simulink library "DevLib"  (R2013b)
settings: Solver=ode45  StartTime=0.0  StopTime=10.0  RelTol=1e-3
undefined symbols (not defined in the file): magnitude, X1, X2, Y1
libraries: simulink x12
settings Model: Creator=HZ69BY  LastModifiedBy=DZ1YRM

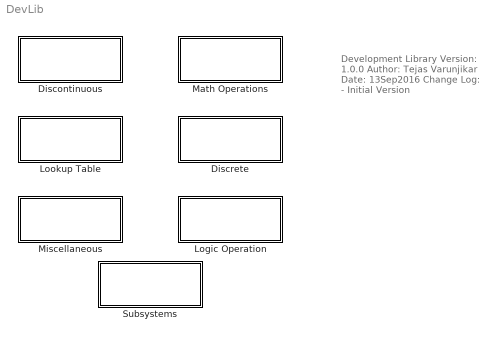
== system DevLib ==
  note: Development Library
      |
      | Version: 1.0.0
      | Author: Tejas Varunjikar
      | Date: 13Sep2016
      | Change Log:
      | - Initial Version
  Discontinuous : Subsystem  mask(Discontinuous){}
      mask Display: fprintf('Discontinuous')
  Discrete : Subsystem
      mask Display: fprintf('Discrete');
  Logic Operation : Subsystem  mask(Logic Operations){}
      mask Display: fprintf('Logic Operation')
  Lookup Table : Subsystem  mask(Lookup Tables){}
      mask Display: fprintf('LookupTable');
  Math Operations : Subsystem  mask(Math Operations){}
      mask Display: fprintf('MathOperations')
  Miscellaneous : Subsystem  mask(Miscellaneous){}
      mask Display: fprintf('Miscellaneous')
  "Subsystems " : Subsystem  mask(Subsystems){}
      mask Display: fprintf('Subsystems')

== system DevLib/Discontinuous ==
  Dead Zone : DeadZone  SaturateOnIntegerOverflow=on
  Dead Zone Dynamic : simulink/Discontinuities/Dead Zone Dynamic
  Rate Limiter : RateLimiter  SampleTimeMode=inherited
  Rate Limiter Dynamic : simulink/Discontinuities/Rate Limiter Dynamic
  Saturation : Saturate
  Saturation Dynamic : simulink/Discontinuities/Saturation Dynamic  OutMin=[]  OutMax=[]  OutDataTypeStr=Inherit: Same as second input  OutDataType=fixdt(1, 16)  OutScaling=2^-10  DoSatur=off

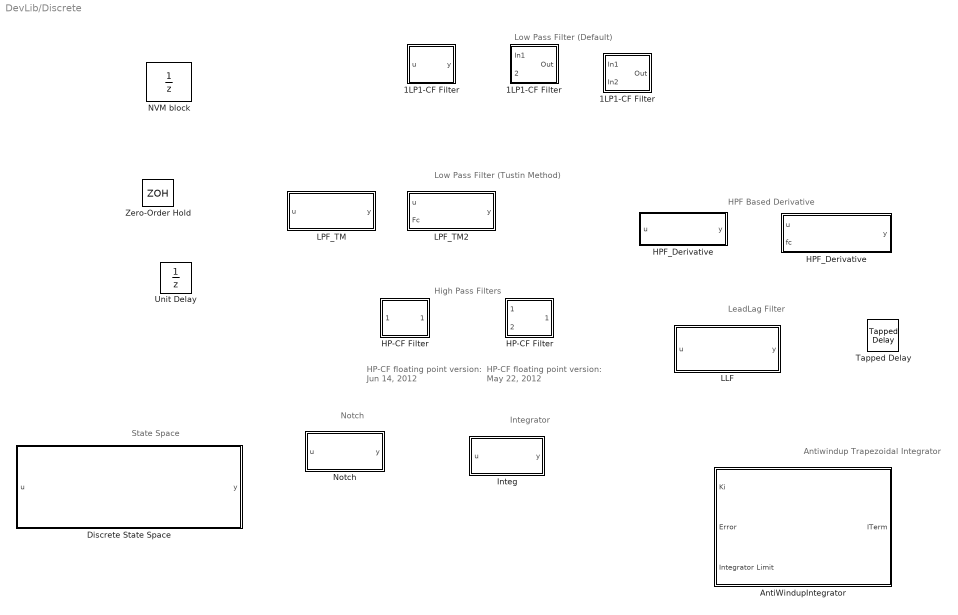
== system DevLib/Discrete ==
  note: HP-CF floating point
      | version:  Jun 14, 2012
  note: HP-CF floating point
      | version:  May 22, 2012
  note: Low Pass Filter (Default)
  note: High Pass Filters
  note: Low Pass Filter (Tustin Method)
  note: Notch
  note: HPF Based Derivative
  note: LeadLag Filter
  note: Integrator
  note: Antiwindup Trapezoidal Integrator
  note: State Space
  " 1LP1-CF Filter " : Subsystem  mask(1LP1-CF Filter){Ts=.002, IC=0}
      mask prompts: Ts "Function Time Step (seconds)"; IC "Initial Condition (Enineering Units)"
      mask help: version: May 22, 2012
      mask Display:
      | port_label('input',1,'u')
      | port_label('input',2,'Hz')
      | port_label('output',1,'y')
      | 
      | %a = [2:0.1:5.2]';
      | %b = sin(2*a);
      | %c = 0.7*sin(25*a);
      | %d = b+c;
      | %e = vertcat(d, b);
      | %plot(e);
      | 
      | disp 'LPF'
  1LP1-CF Filter : Subsystem  mask(1LP1-CF Filter){Ts=.002, Kn_Hz=30, IC=0}
      mask prompts: Ts "Function Time Step (seconds)"; Kn_Hz "Cutoff Frequency in Hz"; IC "Initial Condition (Enineering Units)"
      mask help: version: Jun 14, 2012
      mask init:
      | %Convert cutoff frequency from Hz into floating point "counts"
      | Kn_Cnt = 1-exp(-2*pi*Kn_Hz*Ts);
      | 
      | %Filter design document originally called this value Knum
      | Knum = Kn_Cnt;
      mask Display:
      | port_label('input',1,'u')
      | port_label('output',1,'y')
      | disp 'LPF'
      | 
      | %a = [2:0.1:5.2]';
      | %b = sin(2*a);
      | %c = 0.7*sin(25*a);
      | %d = b+c;
      | %e = vertcat(d, b);
      | %plot(e);
  "1LP1-CF Filter " : Subsystem  mask(1LP1-CF Filter){Ts=.002, Kn_Hz=30}
      mask prompts: Ts "Function Time Step (seconds)"; Kn_Hz "Cutoff Frequency in Hz"
      mask help: version: Aug 31, 2012
      mask init:
      | %Convert cutoff frequency from Hz into floating point "counts"
      | Kn_Cnt = 1-exp(-2*pi*Kn_Hz*Ts);
      | 
      | %Filter design document originally called this value Knum
      | Knum = Kn_Cnt;
      mask Help:
      | 1st order floating point low-pass filter, designated within Nexteer as 1LP1-CF.
      | 
      | This block is arranged to use an externally supplied state variable.  The filter
      | is initialized to the state variable's I.C.
      mask Display:
      | port_label('input',1,'u')
      | port_label('input',2,'sv')
      | port_label('output',1,'y')
      | 
      | disp 'LPF'
  AntiWindupIntegrator : Subsystem  mask(Antiwindup Integrator){Ts=0.002, AntiWdupGain=0}
      mask prompts: Ts "Sample Time"; AntiWdupGain "Anti windup Gain"
      mask help: This is a standard antiwindup integrator design typically used.
      mask Display:
      | fprintf('Antiwindup Integrator');
      | port_label('input',1,'Ki')
      | port_label('input',2,'Error')
      | port_label('input',3,'Integrator Limit')
      | port_label('output',1,'I_term')
  Discrete State Space : Subsystem  mask(Discrete State Space){MtrxA=1, MtrxB=1, MtrxC=1, MtrxD=0, Ts=0.002}
      mask prompts: MtrxA "A"; MtrxB "B"; MtrxC "C"; MtrxD "D"
      mask help:
      | Discrete State Space block representation. Please enter value of state-space matrices. Input, u, is the actuation input to the plant and output, y, is measured state (plant) or estimated state (observer).
      | Input (u) and output (y) could be vectors or single numbers.
      mask Display:
      | fprintf('Discrete State Space');
      | port_label('input',1,'Input')
      | port_label('output',1,'Output')
  HP-CF Filter : Subsystem  mask(HP-CF Filter){Ts_sec=0.002, Fc_Hz=50, LP_IC=0}
      mask prompts: Ts_sec "Function Time Step (seconds)"; Fc_Hz "Cutoff Frequency in Hz"; LP_IC "Input Signal Initial Condition (Engineering Units)"
      mask help: version: June 14, 2012
      mask init:
      | % Correction factor (to be multiplied with HP part)
      | g=2*pi*Fc_Hz*Ts_sec;
      | K=sqrt(1+(2*Fc_Hz*Ts_sec)^2);
      | 
      | corr_factor=(1+exp(g))/(2*K);
      mask Display:
      | port_label('input',1,'y')
      | disp 'HPF'
      | 
      | %a = [2:0.1:5.2]';
      | %b = sin(2*a);
      | %c = 0.5*sin(25*a);
      | %d = b+c;
      | %e = vertcat(d, c);
      | %plot(e);
  "HP-CF Filter " : Subsystem  mask(HP-CF Filter){Ts_sec=0.002, LP_IC=0}
      mask prompts: Ts_sec "Function Time Step (seconds)"; LP_IC "Input Signal Initial Condition (Engineering Units)"
      mask help: version: May 22, 2012
      mask init:
      | g = 2*pi*Ts_sec;
      mask Display:
      | port_label('input',1,'y')
      | port_label('input',2,'Hz')
      | 
      | %a = [2:0.1:5.2]';
      | %b = sin(2*a);
      | %c = 0.5*sin(25*a);
      | %d = b+c;
      | %e = vertcat(d, c);
      | %plot(e);
      | 
      | disp 'HPF'
  HPF_Derivative : Subsystem  mask(High Pass Filter Derivative){Fc=10, Ts=0.002}
      mask prompts: Fc "Cutoff Frequency (Hz)"; Ts "Sample Time"
      mask init:
      | TermN=1-Ts*pi*Fc;
      | TermD=1/(1+Ts*pi*Fc);
      | UnityTerm=2*pi*Fc;
      mask Display: fprintf('HPF Derivative')
  "HPF_Derivative " : Subsystem  mask(HPF Derivative){Ts=0.002}
      mask prompts: Ts "Sample Time"
      mask help: Version June 2, 2016
      mask Display:
      | fprintf('HPF Derivative');
      | port_label('input',1,'u')
      | port_label('input',2,'Fc')
      | port_label('output',1,'y')
  Integ : Subsystem  mask(Integrator){Ki=1, Ts=0.002}
      mask prompts: Ki "Integrator Gain"; Ts "Sample Time"
      mask help:
      | Version: June 2, 2016
      | Digital integrator block representing transfer function Ki/s.
      | Ki is integrator gain.
      mask init:
      | % Initial value of a 1/z variable
      | init1=0;
      mask Display: fprintf('Integrator');
  LLF : Subsystem  mask(Lead Lag Filter){B0=0, B1=0, A1=1, Ts=0.002, Init=0}
      mask prompts: Ts "Sample Time"; Init "State Initialization"
      mask help:
      | Version: June 2, 2016
      | Filter coefficients (B0,B1,A1) of a Lead Lag Filter.
      mask Display:
      | port_label('input',1,'u')
      | port_label('output',1,'y')
      | disp 'LLF'
  LPF_TM : Subsystem  mask{Ts=0.002, fc=1}
      mask prompts: Ts "Sample Time"; fc "Cutoff Frequency"
      mask help:
      | This is a special type of Low Pass Filter.
      | It is designed using tustin transformation method.
      mask Display:
      | fprintf('LPF #2');
      | port_label('input',1,'u')
      | port_label('output',1,'y')
  "LPF_TM2 " : Subsystem  mask{Ts=0.002}
      mask prompts: Ts "Sample Time"
      mask help:
      | This is a special type of Low Pass Filter.
      | It is designed using tustin transformation method.
      mask init:
      | init1=0;
      | init2=0;
      mask Display:
      | fprintf('LPF #2');
      | port_label('input',1,'u')
      | port_label('input',2,'Fc')
      | port_label('output',1,'y')
  NVM block : UnitDelay  SampleTime=-1
      mask help: NVM (Non-volatile memory) block stores a state through ignition cycles.
      mask Display: fprintf('NVM');
  Notch : Subsystem  mask(Notch Filter){A1=0, A2=0, B0=1, B1=0, B2=0, Ts=0.002}
      mask prompts: Ts "Sample time"
      mask help:
      | version: June 2, 2016
      | Numerator (B0,B1,B2) and denominator (1,A1,A2) coefficients of 2nd order digital filter.
      mask init:
      | %Initial values of 2 1/z variables.
      | init1=0;
      | init2=0;
      mask Display: fprintf('Notch Filter')
  Tapped Delay : simulink/Discrete/Tapped Delay  vinit=0.0  samptime=-1  NumDelays=4  DelayOrder=Oldest  includeCurrent=off
  Unit Delay : UnitDelay  SampleTime=-1
  Zero-Order Hold : ZeroOrderHold

== system DevLib/Logic Operation ==
  note: Note: Various logical operators (AND, OR,.. etc. with multiple inputs allowed).
  Action Subsystem : Subsystem  TreatAsAtomicUnit=on
  Bitwise Operator : simulink/Logic and Bit Operations/Bitwise Operator  logicop=AND  UseBitMask=on  BitMask=bin2dec('11011001')  BitMaskRealWorld=Stored Integer
  Compare To Constant : simulink/Logic and Bit Operations/Compare To Constant  relop=<=  const=3.0  OutDataTypeStr=boolean
  Compare To Zero : simulink/Logic and Bit Operations/Compare To Zero  relop=<=  OutDataTypeStr=boolean
  For Iterator Subsystem : Subsystem  TreatAsAtomicUnit=on
  If : If  NumInputs=2  IfExpression=u1  ElseIfExpressions=u2
  Logical Operator : Logic  AllPortsSameDT=off  OutDataTypeStr=boolean
  Merge : Merge  Inputs=3
  Pass through Action Subsystem : Subsystem  TreatAsAtomicUnit=on  mask(pass thru, version Nov 30, 2012){nIn=1}
      mask prompts: nIn "Number of input signals"
      mask help:
      | This block passes its input straight through without modification.
      |
      | Enter the number of signals to pass through (integer 1 to 5).
      mask Callback nIn:
      | thisBlock = gcb;
      | a = get_param(thisBlock,'MaskValues');
      | b = cell2mat(a);
      | c = str2num(b);
      | 
      | if c<1 c=1; end
      | if c>5 c=5; end
      | 
      | for idx=1:c
      |     sIdx = num2str(idx);
      |     oldblock = [thisBlock '/In' sIdx];
      |     if strcmp(get_param(oldblock,'BlockType'),'Ground')
      |          newblock = 'built-in/Inport';
      |         pos = get_param(oldblock,'Position');
      |         orient = get_param(oldblock,'Orientation');
      |         delete_block(oldblock);
      |         add_block(newblock,oldblock,'Position',pos, 'Orientation',orient);
      |     end
      | 
      |     oldblock = [thisBlock '/Out' sIdx];
      |     if strcmp(get_param(oldblock,'BlockType'),'Terminator')
      |         newblock = 'built-in/Outport';
      |         pos = get_param(oldblock,'Position');
      |         orient = get_param(oldblock,'Orientation');
      |         delete_block(oldblock);
      |         add_block(newblock,oldblock,'Position',pos, 'Orientation',orient);
      |     end
      | end
      | 
      | for idx=c+1:5
      |     sIdx = num2str(idx);
      |     oldblock = [thisBlock '/In' sIdx];
      |     if strcmp(get_param(oldblock,'BlockType'),'Inport')
      |         newblock = 'built-in/Ground';
      |         pos = get_param(oldblock,'Position');
      |         orient = get_param(oldblock,'Orientation');
      |         delete_block(oldblock);
      |         add_block(newblock,oldblock,'Position',pos, 'Orientation',orient);
      |     end
      | 
      |     oldblock = [thisBlock '/Out' sIdx];
      |     if strcmp(get_param(oldblock,'BlockType'),'Outport')
      |         newblock = 'built-in/Terminator';
      |         pos = get_param(oldblock,'Position');
      |         orient = get_param(oldblock,'Orientation');
      |         delete_block(oldblock);
      |         add_block(newblock,oldblock,'Position',pos, 'Orientation',orient);
      |     end
      | end
      | 
      | 
      | 
      | clear thisBlock oldblock newblock orient pos a b c idx sIdx ;
      mask Display: fprintf('pass\nthru')
  Relational Operator : RelationalOperator  Operator=<=  OutDataTypeStr=boolean
  Switch Case : SwitchCase
  While Iterator Subsystem : Subsystem  TreatAsAtomicUnit=on

== system DevLib/Lookup Table ==
  note: Note: X2 is typically a vehicle speed 1D table.
  1-D Lookup Table : Lookup_n-D  NumberOfTableDimensions=1  BreakpointsForDimension1=[-5:5]  Table=tanh([-5:5])  ExtrapMethod=Clip  InternalRulePriority=Speed  RndMeth=Simplest  InputSameDT=on
      settings: AttributesFormatString=InterpolationMethod=%<InterpMethod>
  1DX_2DY_Lookup : Subsystem  Tag=Blend Fraction (0 to 1)
  2D_Lookup : Subsystem  mask(2-D Lookup Table){}
  Assist Speed2 : Constant  Value=X2
  Assist Speed4 : Constant  Value=X2
  Constant1 : Constant  Value=X1
  Constant2 : Constant  Value=X1
  Constant3 : Constant  Value=Y1
  Constant4 : Constant  Value=Y1
  wires:
  [X1_in] -> 2D_Lookup/1(X_in)
  Assist Speed4/1 -> 2D_Lookup/5(SpdTbl)
  Constant1/1 -> 2D_Lookup/2(2-D Xtbl)
  Constant3/1 -> 2D_Lookup/3(2-D Ytbl)
  [X2_in] -> 2D_Lookup/4(VehSpeed)
  Assist Speed2/1 -> 1DX_2DY_Lookup/5(SpdTbl)
  Constant2/1 -> 1DX_2DY_Lookup/2(1-D Xtbl)
  Constant4/1 -> 1DX_2DY_Lookup/3(2-D Ytbl)
  [X2_in] -> 1DX_2DY_Lookup/4(Speed)
  [X1_in] -> 1DX_2DY_Lookup/1(X_in)

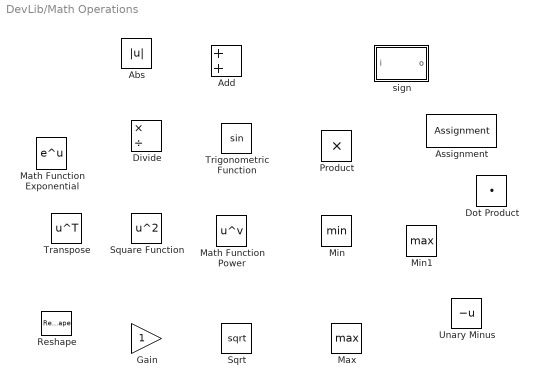
== system DevLib/Math Operations ==
  Abs : Abs
  Add : Sum
  Assignment : Assignment  IndexOptions=Index vector (dialog)  Indices=1  OutputSizes=1
  Divide : Product  Inputs=*/
  Dot Product : DotProduct  InputSameDT=on  OutDataTypeStr=Inherit: Inherit via internal rule
  Gain : Gain
  Math Function Exponential : Math  SaturateOnIntegerOverflow=on
  Math Function Power : Math  Operator=pow  SaturateOnIntegerOverflow=on
  Max : MinMax  Function=max
  Min : MinMax  Inputs=2
  Min1 : MinMax  Function=max  Inputs=2
  Product : Product
  Reshape : Reshape
  Sqrt : Sqrt  SaturateOnIntegerOverflow=on
  Square Function : Math  Operator=square  SaturateOnIntegerOverflow=on
  Transpose : Math  Operator=transpose  SaturateOnIntegerOverflow=on
  Trigonometric Function : Trigonometry
  Unary Minus : UnaryMinus
  sign : Subsystem  mask(2-state sign){}
      mask help:
      | version:  Nov 30, 2012
      |
      | Input < 0, Output = -1
      | Input = 0, Output = +1
      | Input > 0, Output = +1
      mask Help:
      | Input < 0, Output = -1
      | Input = 0, Output = +1
      | Input > 0, Output = +1
      mask Display: disp 'sign'

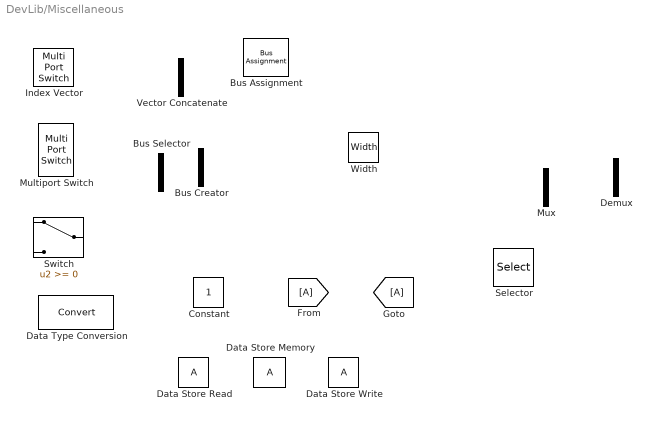
== system DevLib/Miscellaneous ==
  Bus Assignment : BusAssignment  AssignedSignals=signal1
  Bus Creator : BusCreator  Inputs=2
  Bus Selector : BusSelector  OutputSignals=signal1,signal2
  Constant : Constant
  Data Store Memory : DataStoreMemory  ReadBeforeWriteMsg=warning  WriteAfterWriteMsg=warning  WriteAfterReadMsg=warning
  Data Store Read : DataStoreRead
  Data Store Write : DataStoreWrite
  Data Type Conversion : DataTypeConversion
  Demux : Demux  Outputs=2
  Index Vector : MultiPortSwitch  DataPortOrder=Zero-based contiguous  Inputs=1  zeroidx=on
  Multiport Switch : MultiPortSwitch
  Mux : Mux  Inputs=2
  Selector : Selector  InputPortWidth=3  IndexOptions=Index vector (dialog)  Indices=[1 3]  OutputSizes=1
  Switch : Switch
  Vector Concatenate : Concatenate
  Width : Width

== system DevLib/Subsystems  ==
  Enabled Subsystem : Subsystem  TreatAsAtomicUnit=on
  Enabled and Triggered Subsystem : Subsystem  TreatAsAtomicUnit=on
  Function-Call Subsystem : Subsystem  TreatAsAtomicUnit=on
  Subsystem : Subsystem
  Triggered Subsystem : Subsystem  TreatAsAtomicUnit=on
  Variant Subsystem : Subsystem  Variant=on

== system DevLib/Discrete/ 1LP1-CF Filter  ==
  note: Filter layout from spreadsheet
  note: This Subsystem represents a type 1LP1-CF Low-Pass filter with floating point math.
      | Layout and nomenclature taken from Design Document authored by Mark Colosky.
  note: REVISIONS
      |   Feb 13, 2012.  Date created.
      |   Feb 17, 2012.  Conversion from Hz to Knum moved to Initialization tab of mask dialog box.
      |   Feb 20, 2012.  Parameterized 1/z block Initial Condition instead of hard-coded = 0.
      |   May 22, 2012.  Added external cutoff frequency signal.
  In1 : Inport
  KnHz : Inport  Port=2
  Constant : Constant
  Constant1 : Constant  Value=-2*pi*Ts
  Integer Delay : Delay  DelayLength=1  InitialCondition=IC  SampleTime=Ts
  Math Function : Math  SaturateOnIntegerOverflow=on
  Product1 : Product  RndMeth=Zero
  Product2 : Product  RndMeth=Zero
  Subtract : Sum  Inputs=+-
  Sum : Sum  Inputs=|+-
  Sum1 : Sum  Inputs=|++
  Out : Outport
  wires:
  Subtract/1 -> Product1/1
  Product2/1 -> Math Function/1
  KnHz/1 -> Product2/2
  Constant1/1 -> Product2/1
  Math Function/1 -> Subtract/2
  Constant/1 -> Subtract/1
  Sum1/1 -> Out/1, Integer Delay/1  "e"
  In1/1 -> Sum/1  "Unfiltered_Signal"
  Integer Delay/1 -> Sum/2, Sum1/2  "f"
  Product1/1 -> Sum1/1  "d"
  Sum/1 -> Product1/2  "c"

== system DevLib/Discrete/1LP1-CF Filter ==
  note: REVISIONS
      |   Feb 13, 2012.  Date created.
      |   Feb 17, 2012.  Conversion from Hz to Knum moved to Initialization tab of mask dialog box.
      |   Feb 20, 2012.  Parameterized 1/z block Initial Condition instead of hard-coded = 0.
      |   Jun 14, 2012.  Edited Icon to match other 1LP1-CF variants.
  note: This Subsystem represents a type 1LP1-CF Low-Pass filter with floating point math. Layout and nomenclature taken from Design Document authored by Mark Colosky.
  note: Filter layout from spreadsheet
  u : Inport
  Constant : Constant  Value=Knum
  Integer Delay : Delay  DelayLength=1  InitialCondition=IC  SampleTime=Ts
  Product1 : Product  RndMeth=Zero
  Sum : Sum  Inputs=|+-
  Sum1 : Sum  Inputs=|++
  y : Outport
  wires:
  Sum/1 -> Product1/2  "c"
  Constant/1 -> Product1/1
  Product1/1 -> Sum1/1  "d"
  Integer Delay/1 -> Sum1/2, Sum/2  "f"
  u/1 -> Sum/1  "Unfiltered_Signal"
  Sum1/1 -> Integer Delay/1, y/1  "e"

== system DevLib/Discrete/1LP1-CF Filter  ==
  note: REVISIONS
      |   Jun 14, 2012.  Date created.
      |   Aug 31, 2012.  Removed "IC" parameter from mask dialog because it is unused.
      |                            Added information to Help section of mask dialog.
  note: This Subsystem represents a type 1LP1-CF Low-Pass filter with floating point math. Layout and nomenclature taken from Design Document authored by Mark Colosky.
  note: Filter layout from spreadsheet
  In1 : Inport
  In2 : Inport  Port=2
  Constant : Constant  Value=Knum
  Product1 : Product  RndMeth=Zero
  Sum : Sum  Inputs=|+-
  Sum1 : Sum  Inputs=|++
  Out : Outport
  wires:
  In2/1 -> Sum1/2, Sum/2  "f"
  Sum/1 -> Product1/2  "c"
  Constant/1 -> Product1/1
  Product1/1 -> Sum1/1  "d"
  In1/1 -> Sum/1  "Unfiltered_Signal"
  Sum1/1 -> Out/1  "e"

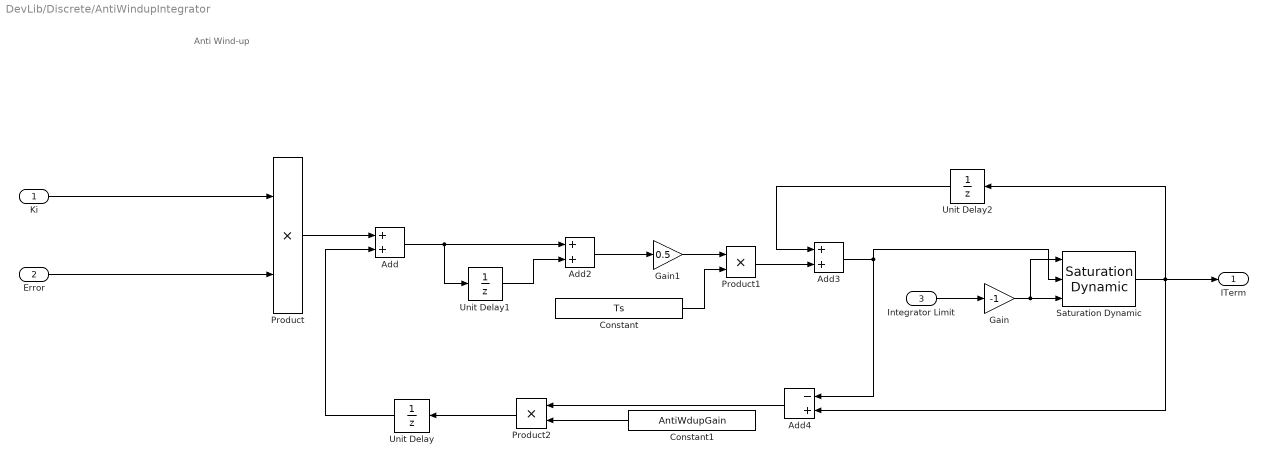
== system DevLib/Discrete/AntiWindupIntegrator ==
  note: Anti Wind-up
  Ki : Inport
  Error : Inport  Port=2
  Integrator Limit : Inport  Port=3
  Add : Sum
  Add2 : Sum
  Add3 : Sum
  Add4 : Sum  Inputs=-+
  Constant : Constant  Value=Ts
  Constant1 : Constant  Value=AntiWdupGain
  Gain : Gain  Gain=-1
  Gain1 : Gain  Gain=0.5
  Product : Product
  Product1 : Product
  Product2 : Product
  Saturation Dynamic : simulink/Discontinuities/Saturation Dynamic  OutMin=[]  OutMax=[]  OutDataTypeStr=Inherit: Same as second input  OutDataType=fixdt(1, 16)  OutScaling=2^-10  DoSatur=off
  Unit Delay : UnitDelay  SampleTime=-1
  Unit Delay1 : UnitDelay  SampleTime=-1
  Unit Delay2 : UnitDelay  SampleTime=-1
  ITerm : Outport
  wires:
  Ki/1 -> Product/1
  Error/1 -> Product/2
  Product/1 -> Add/1
  Unit Delay/1 -> Add/2
  Unit Delay1/1 -> Add2/2
  Add/1 -> Unit Delay1/1, Add2/1
  Add2/1 -> Gain1/1
  Gain1/1 -> Product1/1
  Constant/1 -> Product1/2
  Product1/1 -> Add3/2
  Add3/1 -> Saturation Dynamic/2, Add4/1
  Add4/1 -> Product2/1
  Constant1/1 -> Product2/2
  Product2/1 -> Unit Delay/1
  Saturation Dynamic/1 -> ITerm/1, Unit Delay2/1, Add4/2
  Integrator Limit/1 -> Gain/1
  Unit Delay2/1 -> Add3/1
  Gain/1 -> Saturation Dynamic/1, Saturation Dynamic/3

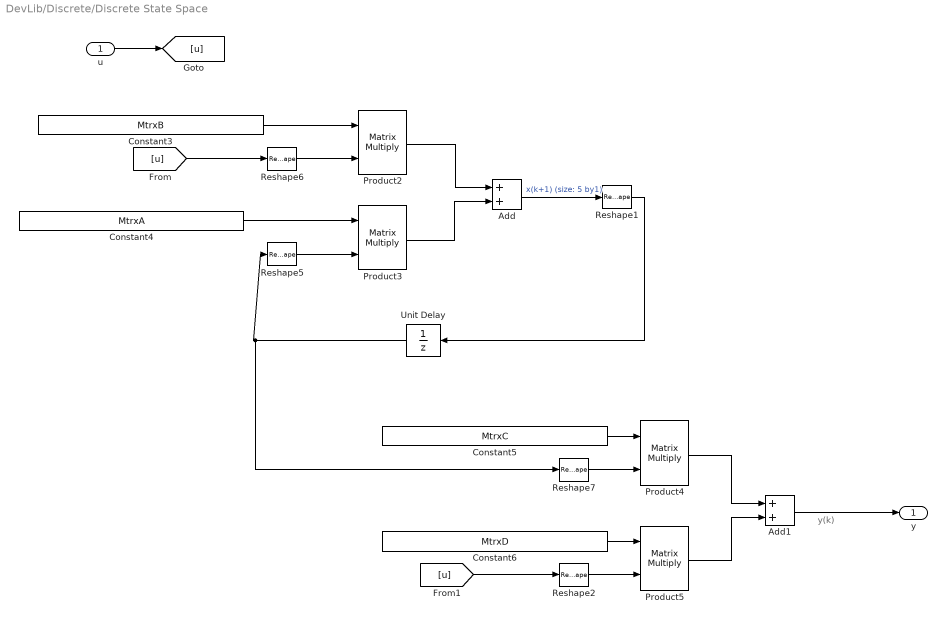
== system DevLib/Discrete/Discrete State Space ==
  note: y(k)
  u : Inport  RequirementInfo={'linktype_rmi_doors' '000126ea (/E-STEER Core/SubSystem Specifications/Application Functions/SF056A Driver Torque Estimation)' '#SF056A_31' 'true' 'REQ:SF056A_31' '' } %GIDa_36e1b196_1e9c_4edd_90d4_32c470667677
  Add : Sum  RequirementInfo={'linktype_rmi_doors' '000126ea (/E-STEER Core/SubSystem Specifications/Application Functions/SF056A Driver Torque Estimation)' '#SF056A_31' 'true' 'REQ:SF056A_31' '' } %GIDa_d9b928e3_ce52_494d_9c1d_07750e97f849
  Add1 : Sum  RequirementInfo={'linktype_rmi_doors' '000126ea (/E-STEER Core/SubSystem Specifications/Application Functions/SF056A Driver Torque Estimation)' '#SF056A_33' 'true' 'REQ:SF056A_33' '' } %GIDa_7d255f73_6f23_4e2d_bfae_e4de095026f1
  Constant3 : Constant  RequirementInfo={'linktype_rmi_doors' '000126ea (/E-STEER Core/SubSystem Specifications/Application Functions/SF056A Driver Torque Estimation)' '#SF056A_31' 'true' 'REQ:SF056A_31' '' } %GIDa_8b31cdbd_4cc1_41b4_9c17_828c8857f523  Value=MtrxB
  Constant4 : Constant  RequirementInfo={'linktype_rmi_doors' '000126ea (/E-STEER Core/SubSystem Specifications/Application Functions/SF056A Driver Torque Estimation)' '#SF056A_31' 'true' 'REQ:SF056A_31' '' } %GIDa_7b20900d_6959_4fd1_b2b3_a76fa8c068f6  Value=MtrxA  VectorParams1D=off
  Constant5 : Constant  RequirementInfo={'linktype_rmi_doors' '000126ea (/E-STEER Core/SubSystem Specifications/Application Functions/SF056A Driver Torque Estimation)' '#SF056A_33' 'true' 'REQ:SF056A_33' '' } %GIDa_009ff853_244d_4f28_ba80_168666defd5a  Value=MtrxC  VectorParams1D=off
  Constant6 : Constant  RequirementInfo={'linktype_rmi_doors' '000126ea (/E-STEER Core/SubSystem Specifications/Application Functions/SF056A Driver Torque Estimation)' '#SF056A_33' 'true' 'REQ:SF056A_33' '' } %GIDa_417dab65_9bd6_4e2c_8260_53ef8aa46bcf  Value=MtrxD  VectorParams1D=off
  Product2 : Product  RequirementInfo={'linktype_rmi_doors' '000126ea (/E-STEER Core/SubSystem Specifications/Application Functions/SF056A Driver Torque Estimation)' '#SF056A_31' 'true' 'REQ:SF056A_31' '' } %GIDa_c519823f_36d5_49cb_97a7_0803cded37c3  Multiplication=Matrix(*)
  Product3 : Product  RequirementInfo={'linktype_rmi_doors' '000126ea (/E-STEER Core/SubSystem Specifications/Application Functions/SF056A Driver Torque Estimation)' '#SF056A_31' 'true' 'REQ:SF056A_31' '' } %GIDa_fb90a766_6c5c_4856_b7d9_2bbb42394132  Multiplication=Matrix(*)
  Product4 : Product  RequirementInfo={'linktype_rmi_doors' '000126ea (/E-STEER Core/SubSystem Specifications/Application Functions/SF056A Driver Torque Estimation)' '#SF056A_33' 'true' 'REQ:SF056A_33' '' } %GIDa_da78b708_0780_4ea0_8037_183ecda744fd  Multiplication=Matrix(*)
  Product5 : Product  RequirementInfo={'linktype_rmi_doors' '000126ea (/E-STEER Core/SubSystem Specifications/Application Functions/SF056A Driver Torque Estimation)' '#SF056A_33' 'true' 'REQ:SF056A_33' '' } %GIDa_b433201e_1314_49bc_894b_46f00e689d1d  Multiplication=Matrix(*)
  Reshape{1..2,5..7} (5 alike) : Reshape  OutputDimensionality=Column vector (2-D)
  Unit Delay : UnitDelay  SampleTime=Ts
  y : Outport  RequirementInfo={'linktype_rmi_doors' '000126ea (/E-STEER Core/SubSystem Specifications/Application Functions/SF056A Driver Torque Estimation)' '#SF056A_33' 'true' 'REQ:SF056A_33' '' } %GIDa_dd02f87e_4347_4cfa_9b3c_8c1400debd29
  wires:
  [u] -> Reshape6/1
  Constant3/1 -> Product2/1
  Constant4/1 -> Product3/1
  Product2/1 -> Add/1
  Product3/1 -> Add/2
  Add/1 -> Reshape1/1  "x(k+1) (size: 5 by1)"
  Constant5/1 -> Product4/1
  Unit Delay/1 -> Reshape7/1, Reshape5/1
  Constant6/1 -> Product5/1
  [u] -> Reshape2/1
  Product4/1 -> Add1/1
  Product5/1 -> Add1/2
  Add1/1 -> y/1
  u/1 -> [u]
  Reshape1/1 -> Unit Delay/1
  Reshape5/1 -> Product3/2
  Reshape6/1 -> Product2/2
  Reshape7/1 -> Product4/2
  Reshape2/1 -> Product5/2

== system DevLib/Discrete/HP-CF Filter ==
  note: HP filtered signal = (Raw Signal - LP filtered signal) * correction factor
      |
      | Low-pass filter is type 1LP1-CF floating point.
      | Correction factor accounts for error caused by discrete implementation.
  note: REVISIONS
      |   Mar 05, 2012.  Date created.
      |   Mar 16, 2012.  corr_factor changed.  (see mask initialization).
      |   Jun 14, 2012.  Changed icon to match other floating-point variants.
  note: This Subsystem represents a high-pass floating point filter.
  Input : Inport
  1LP1-CF Filter : Subsystem  mask(1LP1-CF Filter){Ts=.002, Kn_Hz=30, IC=0}
      mask prompts: Ts "Function Time Step (seconds)"; Kn_Hz "Cutoff Frequency in Hz"; IC "Initial Condition (Enineering Units)"
      mask help: version: Jun 14, 2012
      mask init:
      | %Convert cutoff frequency from Hz into floating point "counts"
      | Kn_Cnt = 1-exp(-2*pi*Kn_Hz*Ts);
      | 
      | %Filter design document originally called this value Knum
      | Knum = Kn_Cnt;
      mask Display:
      | port_label('input',1,'y')
      | disp 'LPF'
      | 
      | %a = [2:0.1:5.2]';
      | %b = sin(2*a);
      | %c = 0.7*sin(25*a);
      | %d = b+c;
      | %e = vertcat(d, b);
      | %plot(e);
  Correction_factor : Constant  Value=corr_factor  OutDataTypeStr=Inherit: Inherit via back propagation
  Product : Product  RndMeth=Zero
  Sum : Sum  Inputs=|+-
  Output : Outport
  wires:
  Input/1 -> Sum/1, 1LP1-CF Filter/1(In1)  "Unfiltered_Signal"
  1LP1-CF Filter/1(Out) -> Sum/2  "filtered_LP_Part"
  Sum/1 -> Product/1
  Correction_factor/1 -> Product/2
  Product/1 -> Output/1  "corrected_HP_part"

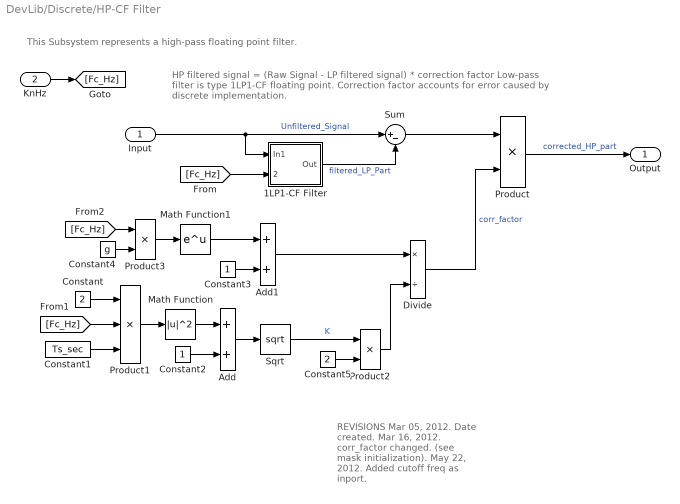
== system DevLib/Discrete/HP-CF Filter  ==
  note: This Subsystem represents a high-pass floating point filter.
  note: REVISIONS
      |   Mar 05, 2012.  Date created.
      |   Mar 16, 2012.  corr_factor changed.  (see mask initialization).
      |   May 22, 2012.  Added cutoff freq as inport.
  note: HP filtered signal = (Raw Signal - LP filtered signal) * correction factor
      |
      | Low-pass filter is type 1LP1-CF floating point.
      | Correction factor accounts for error caused by discrete implementation.
  Input : Inport
  KnHz : Inport  Port=2
  1LP1-CF Filter : Subsystem  mask(1LP1-CF Filter){Ts=.002, IC=0}
      mask prompts: Ts "Function Time Step (seconds)"; IC "Initial Condition (Enineering Units)"
      mask help: version: May 22, 2012
      mask Display:
      | port_label('input',1,'y')
      | port_label('input',2,'Hz')
      | 
      | %a = [2:0.1:5.2]';
      | %b = sin(2*a);
      | %c = 0.7*sin(25*a);
      | %d = b+c;
      | %e = vertcat(d, b);
      | %plot(e);
      | 
      | disp 'LPF'
  Add : Sum
  Add1 : Sum
  Constant : Constant  Value=2  OutDataTypeStr=Inherit: Inherit via back propagation
  Constant1 : Constant  Value=Ts_sec  OutDataTypeStr=Inherit: Inherit via back propagation
  Constant2 : Constant  OutDataTypeStr=Inherit: Inherit via back propagation
  Constant3 : Constant
  Constant4 : Constant  Value=g  OutDataTypeStr=Inherit: Inherit via back propagation
  Constant5 : Constant  Value=2  OutDataTypeStr=Inherit: Inherit via back propagation
  Divide : Product  Inputs=*/
  Math Function : Math  Operator=magnitude^2  SaturateOnIntegerOverflow=on
  Math Function1 : Math  SaturateOnIntegerOverflow=on
  Product : Product  RndMeth=Zero
  Product1 : Product  Inputs=3  RndMeth=Zero
  Product2 : Product  RndMeth=Zero
  Product3 : Product  RndMeth=Zero
  Sqrt : Sqrt  SaturateOnIntegerOverflow=on
  Sum : Sum  Inputs=|+-
  Output : Outport
  wires:
  Divide/1 -> Product/2  "corr_factor"
  Product2/1 -> Divide/2
  Add1/1 -> Divide/1
  Constant1/1 -> Product1/3
  [Fc_Hz] -> Product1/2
  Constant4/1 -> Product3/2
  [Fc_Hz] -> Product3/1
  Product3/1 -> Math Function1/1
  Constant5/1 -> Product2/2
  Sqrt/1 -> Product2/1  "K"
  Math Function1/1 -> Add1/1
  Constant3/1 -> Add1/2
  Add/1 -> Sqrt/1
  Constant2/1 -> Add/2
  Math Function/1 -> Add/1
  Product1/1 -> Math Function/1
  KnHz/1 -> [Fc_Hz]
  Constant/1 -> Product1/1
  Product/1 -> Output/1  "corrected_HP_part"
  Sum/1 -> Product/1
  1LP1-CF Filter/1(Out) -> Sum/2  "filtered_LP_Part"
  Input/1 -> 1LP1-CF Filter/1(In1), Sum/1  "Unfiltered_Signal"
  [Fc_Hz] -> 1LP1-CF Filter/2(KnHz)

== system DevLib/Discrete/HPF_Derivative ==
  u : Inport
  Constant6 : Constant  Value=TermD
  Constant7 : Constant  Value=TermN
  Constant8 : Constant  Value=UnityTerm
  Product1 : Product
  Product3 : Product
  Product4 : Product
  Sum4 : Sum  Inputs=|+-
  Sum7 : Sum  Inputs=|++
  Unit Delay1 : UnitDelay  SampleTime=-1
  Unit Delay2 : UnitDelay  SampleTime=-1
  y : Outport
  wires:
  Unit Delay1/1 -> Sum4/2
  u/1 -> Sum4/1, Unit Delay1/1
  Constant7/1 -> Product3/1
  Unit Delay2/1 -> Product3/2
  Product4/1 -> Unit Delay2/1, Product1/2
  Product3/1 -> Sum7/2
  Sum4/1 -> Sum7/1
  Constant6/1 -> Product4/1
  Sum7/1 -> Product4/2
  Product1/1 -> y/1
  Constant8/1 -> Product1/1

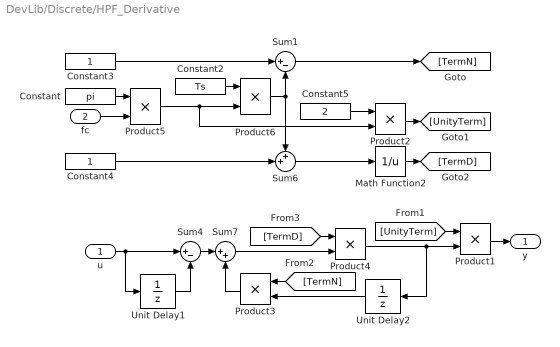
== system DevLib/Discrete/HPF_Derivative  ==
  u : Inport
  fc : Inport  Port=2
  Constant : Constant  Value=pi
  Constant2 : Constant  Value=Ts
  Constant3 : Constant
  Constant4 : Constant
  Constant5 : Constant  Value=2
  Math Function2 : Math  Operator=reciprocal  SaturateOnIntegerOverflow=on
  Product{1..6} (6 alike) : Product
  Sum1 : Sum  Inputs=|+-
  Sum4 : Sum  Inputs=|+-
  Sum6 : Sum  Inputs=++|
  Sum7 : Sum  Inputs=|++
  Unit Delay1 : UnitDelay  SampleTime=-1
  Unit Delay2 : UnitDelay  SampleTime=-1
  y : Outport
  wires:
  Unit Delay1/1 -> Sum4/2
  Constant2/1 -> Product6/1
  fc/1 -> Product5/2
  Constant/1 -> Product5/1
  Constant3/1 -> Sum1/1
  Product6/1 -> Sum6/1, Sum1/2
  Sum1/1 -> [TermN]
  Constant4/1 -> Sum6/2
  Sum6/1 -> Math Function2/1
  Math Function2/1 -> [TermD]
  u/1 -> Sum4/1, Unit Delay1/1
  [TermN] -> Product3/1
  Unit Delay2/1 -> Product3/2
  Product4/1 -> Unit Delay2/1, Product1/2
  Product3/1 -> Sum7/2
  Sum4/1 -> Sum7/1
  [TermD] -> Product4/1
  Sum7/1 -> Product4/2
  Product1/1 -> y/1
  [UnityTerm] -> Product1/1
  Product2/1 -> [UnityTerm]
  Constant5/1 -> Product2/1
  Product5/1 -> Product2/2, Product6/2

== system DevLib/Discrete/Integ ==
  u : Inport
  Constant6 : Constant  Value=Ki
  Constant7 : Constant  Value=Ts
  Product7 : Product  Inputs=3
  Sum2 : Sum  Inputs=|++
  Unit Delay2 : UnitDelay  InitialCondition=init1  SampleTime=-1
  y : Outport
  wires:
  Sum2/1 -> y/1, Unit Delay2/1
  u/1 -> Product7/1
  Constant6/1 -> Product7/2
  Constant7/1 -> Product7/3
  Product7/1 -> Sum2/1
  Unit Delay2/1 -> Sum2/2

== system DevLib/Discrete/LLF ==
  note: When the Temperature Estimation function executes for the first time, the filter output
      | is set to CtrlTemp. The state variable will automatically be initialized.
      |
      | The initialization scheme can be mathematically expressed as follows,
      | y(0) = CtrlTemp;
      | x(0) = A1*y(0) + B1*u(0);
      | where y = output, x = state variable, u = input
      |
      | The general equation for the n-th time-step will be,
      | y(n) = x(n-1) + B0*u(n);
      | x(n) = A1*y(n-1) + B1*u(n-1);
      |
      | Note that if the filter output is initialized (to zero) when the value of CtrlTemp is not stable,
      | the state variable will get initialized to an incorrect value, and will result in grossly incorrect
      | temperature estimates.
      |
      | Note that the filter needs to be re-initialized using the specified method at the beginning of
      | each ignition cycle.
  u : Inport
  Copper Lead Lag Filter A1 : Constant  Value=A1  OutDataTypeStr=Inherit: Inherit via back propagation
  Copper Lead Lag Filter B0 : Constant  Value=B0  OutDataTypeStr=Inherit: Inherit via back propagation
  Copper Lead Lag Filter B1 : Constant  Value=B1  OutDataTypeStr=Inherit: Inherit via back propagation
  Copper Lead Lag Filter B2 : Constant  Value=Init  OutDataTypeStr=Inherit: Inherit via back propagation
  Delay : Delay  DelayLength=1  InitialConditionSource=Input port  SampleTime=Ts
      settings: InputPortMap=u0,p4
  Product (1) : Product  RndMeth=Zero
  Product (2) : Product  RndMeth=Zero
  Product (3) : Product  RndMeth=Zero
  Sum (1) : Sum  Inputs=|++
  Sum (2) : Sum  Inputs=++|
  y : Outport
  wires:
  Copper Lead Lag Filter B0/1 -> Product (1)/2
  Product (2)/1 -> Sum (1)/1
  Copper Lead Lag Filter B1/1 -> Product (2)/1
  Sum (1)/1 -> Delay/1
  Delay/1 -> Sum (2)/2
  Product (1)/1 -> Sum (2)/1
  Product (3)/1 -> Sum (1)/2
  Sum (2)/1 -> y/1, Product (3)/1
  Copper Lead Lag Filter A1/1 -> Product (3)/2
  u/1 -> Product (1)/1, Product (2)/2
  Copper Lead Lag Filter B2/1 -> Delay/2

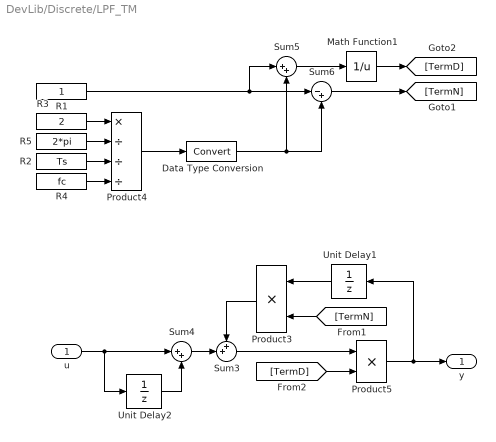
== system DevLib/Discrete/LPF_TM ==
  u : Inport
  Data Type Conversion : DataTypeConversion
  Math Function1 : Math  Operator=reciprocal  SaturateOnIntegerOverflow=on
  Product3 : Product
  Product4 : Product  Inputs=*///
  Product5 : Product  Inputs=**
  R1 : Constant  OutDataTypeStr=Inherit: Inherit via back propagation
  R2 : Constant  Value=Ts  OutDataTypeStr=Inherit: Inherit via back propagation
  R3 : Constant  Value=2  OutDataTypeStr=Inherit: Inherit via back propagation
  R4 : Constant  Value=fc  OutDataTypeStr=Inherit: Inherit via back propagation
  R5 : Constant  Value=2*pi  OutDataTypeStr=Inherit: Inherit via back propagation
  Sum3 : Sum  Inputs=++|
  Sum4 : Sum  Inputs=|++
  Sum5 : Sum  Inputs=|++  OutDataTypeStr=Inherit: Inherit via back propagation
  Sum6 : Sum  Inputs=|-+
  Unit Delay1 : UnitDelay  SampleTime=-1
  Unit Delay2 : UnitDelay  SampleTime=-1
  y : Outport
  wires:
  R3/1 -> Product4/1
  Product3/1 -> Sum3/1
  Unit Delay1/1 -> Product3/1
  u/1 -> Sum4/1, Unit Delay2/1
  Product5/1 -> y/1, Unit Delay1/1
  R2/1 -> Product4/3
  Unit Delay2/1 -> Sum4/2
  Sum4/1 -> Sum3/2
  Sum6/1 -> [TermN]
  [TermN] -> Product3/2
  R4/1 -> Product4/4
  Product4/1 -> Data Type Conversion/1
  R1/1 -> Sum5/1, Sum6/1
  Sum5/1 -> Math Function1/1
  Sum3/1 -> Product5/1
  [TermD] -> Product5/2
  Math Function1/1 -> [TermD]
  R5/1 -> Product4/2
  Data Type Conversion/1 -> Sum6/2, Sum5/2

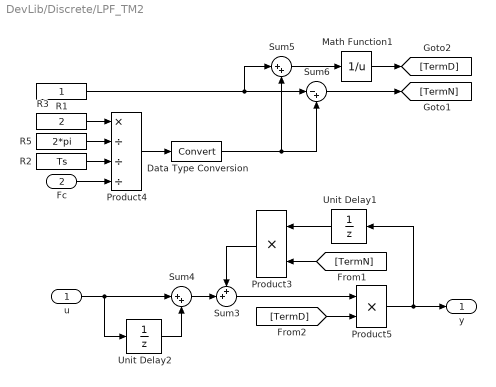
== system DevLib/Discrete/LPF_TM2  ==
  u : Inport
  Fc : Inport  Port=2
  Data Type Conversion : DataTypeConversion
  Math Function1 : Math  Operator=reciprocal  SaturateOnIntegerOverflow=on
  Product3 : Product
  Product4 : Product  Inputs=*///
  Product5 : Product  Inputs=**
  R1 : Constant  OutDataTypeStr=Inherit: Inherit via back propagation
  R2 : Constant  Value=Ts  OutDataTypeStr=Inherit: Inherit via back propagation
  R3 : Constant  Value=2  OutDataTypeStr=Inherit: Inherit via back propagation
  R5 : Constant  Value=2*pi  OutDataTypeStr=Inherit: Inherit via back propagation
  Sum3 : Sum  Inputs=++|
  Sum4 : Sum  Inputs=|++
  Sum5 : Sum  Inputs=|++
  Sum6 : Sum  Inputs=|-+
  Unit Delay1 : UnitDelay  InitialCondition=init2  SampleTime=-1
  Unit Delay2 : UnitDelay  InitialCondition=init1  SampleTime=-1
  y : Outport
  wires:
  R5/1 -> Product4/2
  Math Function1/1 -> [TermD]
  [TermD] -> Product5/2
  Sum3/1 -> Product5/1
  Sum5/1 -> Math Function1/1
  R1/1 -> Sum6/1, Sum5/1
  Product4/1 -> Data Type Conversion/1
  Fc/1 -> Product4/4
  [TermN] -> Product3/2
  Sum6/1 -> [TermN]
  Sum4/1 -> Sum3/2
  Unit Delay2/1 -> Sum4/2
  R2/1 -> Product4/3
  Product5/1 -> Unit Delay1/1, y/1
  u/1 -> Unit Delay2/1, Sum4/1
  Unit Delay1/1 -> Product3/1
  Product3/1 -> Sum3/1
  R3/1 -> Product4/1
  Data Type Conversion/1 -> Sum5/2, Sum6/2

== system DevLib/Discrete/Notch ==
  u : Inport
  Gain : Gain  Gain=B0
  Gain1 : Gain  Gain=A1
  Gain2 : Gain  Gain=B1
  Gain3 : Gain  Gain=B2
  Gain4 : Gain  Gain=A2
  Sum1 : Sum  Inputs=|++
  Sum2 : Sum  Inputs=+-+
  Sum7 : Sum  Inputs=|+-
  Unit Delay3 : UnitDelay  InitialCondition=init2  SampleTime=Ts
  Unit Delay4 : UnitDelay  InitialCondition=init1  SampleTime=Ts
  y : Outport
  wires:
  u/1 -> Gain2/1, Gain3/1, Gain/1
  Gain/1 -> Sum1/1
  Unit Delay3/1 -> Sum1/2
  Sum1/1 -> Gain4/1, Gain1/1, y/1
  Gain1/1 -> Sum2/2
  Gain2/1 -> Sum2/1
  Gain3/1 -> Sum7/1
  Gain4/1 -> Sum7/2
  Sum7/1 -> Unit Delay4/1
  Unit Delay4/1 -> Sum2/3
  Sum2/1 -> Unit Delay3/1  "x"

== system DevLib/Logic Operation/Action Subsystem ==
  In1 : Inport
  Action Port : ActionPort
  Out1 : Outport
  wires:
  In1/1 -> Out1/1

== system DevLib/Logic Operation/For Iterator Subsystem ==
  In1 : Inport
  For Iterator : ForIterator
  Out1 : Outport
  wires:
  In1/1 -> Out1/1

== system DevLib/Logic Operation/Pass through Action Subsystem ==
  note: Change Log:
      | Oct 12, 2012  Created by Kevin Derry as a 1-input, 1-output block
      | Nov 30, 2012  dynamically configurable for 1 to 5 ports.
  note: Do not modify these blocks manually.  They
      | are generated programatically.  Changing the
      | number of blocks available or their names requires
      | corresponding changes to Callback and Initialization
      | routines.
      |
      | Do not change the "Display" tab of mask editor.  The
      | outport names are created programatically in the
      | "Initialize" section.
  In1 : Inport
  Action Port : ActionPort
  In{2..5} (4 alike) : Ground
  Out{2..5} (4 alike) : Terminator
  Out1 : Outport
  wires:
  In1/1 -> Out1/1
  In2/1 -> Out2/1
  In3/1 -> Out3/1
  In4/1 -> Out4/1
  In5/1 -> Out5/1

== system DevLib/Logic Operation/While Iterator Subsystem ==
  In1 : Inport
  IC : Inport  Port=2
  While Iterator : WhileIterator
  Out1 : Outport
  wires:
  IC/1 -> While Iterator/2
  In1/1 -> Out1/1

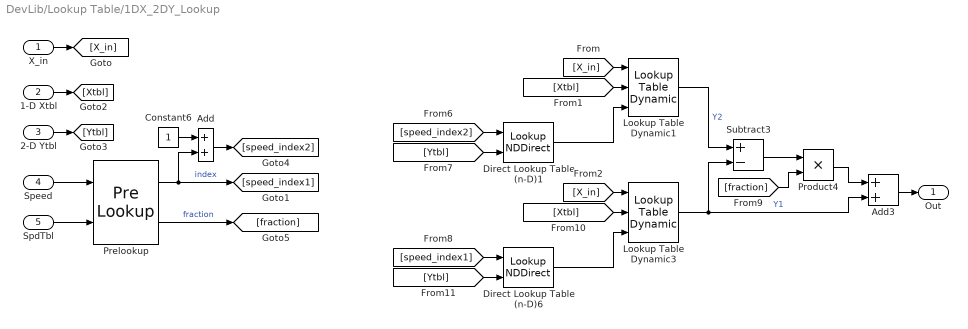
== system DevLib/Lookup Table/1DX_2DY_Lookup ==
  X_in : Inport
  1-D Xtbl : Inport  Port=2
  2-D Ytbl : Inport  Port=3
  Speed : Inport  Port=4
  SpdTbl : Inport  Port=5
  Add : Sum
  Add3 : Sum
  Constant6 : Constant
  Direct Lookup Table (n-D)1 : LookupNDDirect  InputsSelectThisObjectFromTable=Column  TableIsInput=on  DiagnosticForOutOfRangeInput=None
  Direct Lookup Table (n-D)6 : LookupNDDirect  InputsSelectThisObjectFromTable=Column  TableIsInput=on
  Lookup Table Dynamic1 : simulink/Lookup Tables/Lookup Table Dynamic  LookUpMeth=Interpolation-Use End Values  OutDataTypeStr=fixdt('double')  OutputDataTypeScalingMode=Specify via dialog  OutDataType=fixdt('double')  OutScaling=2^-10  DoSatur=off
  Lookup Table Dynamic3 : simulink/Lookup Tables/Lookup Table Dynamic  LookUpMeth=Interpolation-Use End Values  OutDataTypeStr=fixdt('double')  OutputDataTypeScalingMode=Specify via dialog  OutDataType=fixdt('double')  OutScaling=2^-10  DoSatur=off
  Prelookup : PreLookup  BreakpointsDataSource=Input port  BreakpointsData=[10:10:110]  UseLastBreakpoint=on
      settings: InputPortMap=u0,p1
  Product4 : Product  RndMeth=Zero
  Subtract3 : Sum  Inputs=+-
  Out : Outport
  wires:
  Lookup Table Dynamic1/1 -> Subtract3/1  "Y2"
  Subtract3/1 -> Product4/1
  Product4/1 -> Add3/1
  [Ytbl] -> Direct Lookup Table (n-D)1/2
  Direct Lookup Table (n-D)1/1 -> Lookup Table Dynamic1/3
  [X_in] -> Lookup Table Dynamic1/1
  [Ytbl] -> Direct Lookup Table (n-D)6/2
  [Xtbl] -> Lookup Table Dynamic3/2
  Direct Lookup Table (n-D)6/1 -> Lookup Table Dynamic3/3
  [X_in] -> Lookup Table Dynamic3/1
  [speed_index2] -> Direct Lookup Table (n-D)1/1
  [speed_index1] -> Direct Lookup Table (n-D)6/1
  Lookup Table Dynamic3/1 -> Subtract3/2, Add3/2  "Y1"
  [fraction] -> Product4/2
  1-D Xtbl/1 -> [Xtbl]
  2-D Ytbl/1 -> [Ytbl]
  X_in/1 -> [X_in]
  Speed/1 -> Prelookup/1
  Constant6/1 -> Add/1
  Prelookup/1 -> [speed_index1], Add/2  "index"
  Add/1 -> [speed_index2]
  Prelookup/2 -> [fraction]  "fraction"
  SpdTbl/1 -> Prelookup/2
  Add3/1 -> Out/1
  [Xtbl] -> Lookup Table Dynamic1/2

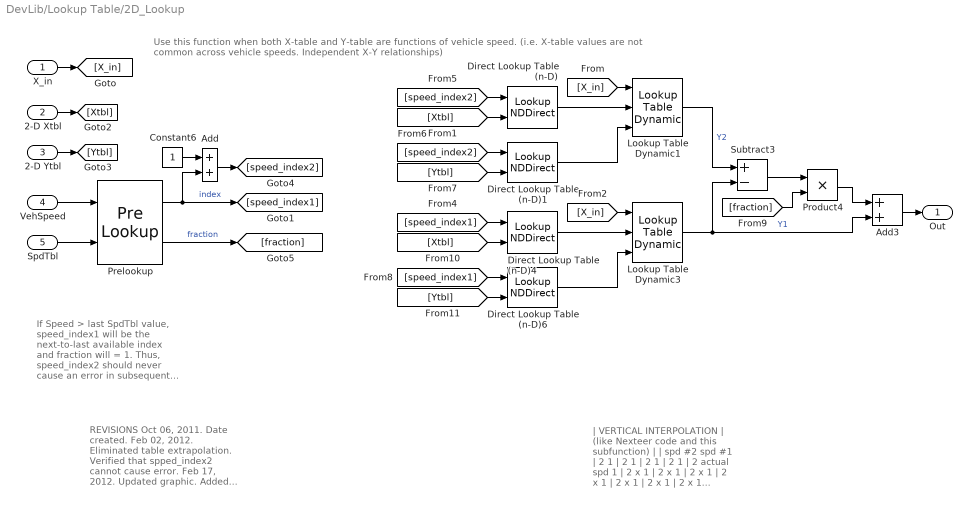
== system DevLib/Lookup Table/2D_Lookup ==
  note: REVISIONS
      |   Oct 06, 2011.  Date created.
      |   Feb 02, 2012.  Eliminated table extrapolation.  Verified that spped_index2 cannot cause error.
      |   Feb 17, 2012.  Updated graphic.  Added this revision block.
      |   Apr  19, 2012.  Renamed Speed to VehSpeed for clarity.
  note: |         VERTICAL INTERPOLATION
      | |                    (like Nexteer code and this subfunction)
      | |
      | |                                        spd #2                    spd #1
      | |                                           2                             1
      | |                                         2                            1
      | |                                       2                           1
      | |                                    2                           1
      | |                                 2     actual spd      1
      | |                              2            x             1
      | |                           2            x            1
      | |                        2            x            1
      | |                    2            x             1
      | |                 2           x             1
      | |            2        x                 1
      | |     2         x                  1
      | |2_x_____________1_____________________________
  note: Use this function when both X-table and Y-table are functions of vehicle speed.
      | (i.e. X-table values are not common across vehicle speeds.  Independent X-Y relationships)
  note: If Speed > last SpdTbl value, speed_index1 will be the
      | next-to-last available index and fraction will = 1.  Thus,
      | speed_index2 should never cause an error in subsequent
      | lookup tables.
  X_in : Inport
  2-D Xtbl : Inport  Port=2
  2-D Ytbl : Inport  Port=3
  VehSpeed : Inport  Port=4
  SpdTbl : Inport  Port=5
  Add : Sum
  Add3 : Sum
  Constant6 : Constant
  Direct Lookup Table (n-D){,1,4,6} (4 alike) : LookupNDDirect  InputsSelectThisObjectFromTable=Column  TableIsInput=on
  Lookup Table Dynamic1 : simulink/Lookup Tables/Lookup Table Dynamic  LookUpMeth=Interpolation-Use End Values  OutDataTypeStr=fixdt('double')  OutputDataTypeScalingMode=Specify via dialog  OutDataType=fixdt('double')  OutScaling=2^-10  DoSatur=off
  Lookup Table Dynamic3 : simulink/Lookup Tables/Lookup Table Dynamic  LookUpMeth=Interpolation-Use End Values  OutDataTypeStr=fixdt('double')  OutputDataTypeScalingMode=Specify via dialog  OutDataType=fixdt('double')  OutScaling=2^-10  DoSatur=off
  Prelookup : PreLookup  BreakpointsDataSource=Input port  BreakpointsData=[10:10:110]
      settings: InputPortMap=u0,p1
  Product4 : Product  RndMeth=Zero
  Subtract3 : Sum  Inputs=+-
  Out : Outport
  wires:
  Add3/1 -> Out/1
  SpdTbl/1 -> Prelookup/2
  Prelookup/2 -> [fraction]  "fraction"
  Add/1 -> [speed_index2]
  Prelookup/1 -> Add/2, [speed_index1]  "index"
  Constant6/1 -> Add/1
  VehSpeed/1 -> Prelookup/1
  X_in/1 -> [X_in]
  2-D Ytbl/1 -> [Ytbl]
  2-D Xtbl/1 -> [Xtbl]
  [fraction] -> Product4/2
  Lookup Table Dynamic3/1 -> Add3/2, Subtract3/2  "Y1"
  [speed_index1] -> Direct Lookup Table (n-D)6/1
  [speed_index1] -> Direct Lookup Table (n-D)4/1
  [speed_index2] -> Direct Lookup Table (n-D)1/1
  [speed_index2] -> Direct Lookup Table (n-D)/1
  [X_in] -> Lookup Table Dynamic3/1
  Direct Lookup Table (n-D)6/1 -> Lookup Table Dynamic3/3
  Direct Lookup Table (n-D)4/1 -> Lookup Table Dynamic3/2
  [Ytbl] -> Direct Lookup Table (n-D)6/2
  [Xtbl] -> Direct Lookup Table (n-D)4/2
  [X_in] -> Lookup Table Dynamic1/1
  Direct Lookup Table (n-D)1/1 -> Lookup Table Dynamic1/3
  Direct Lookup Table (n-D)/1 -> Lookup Table Dynamic1/2
  [Ytbl] -> Direct Lookup Table (n-D)1/2
  [Xtbl] -> Direct Lookup Table (n-D)/2
  Product4/1 -> Add3/1
  Subtract3/1 -> Product4/1
  Lookup Table Dynamic1/1 -> Subtract3/1  "Y2"

== system DevLib/Math Operations/sign ==
  note: REVISIONS
      |   Jan 31, 2012.  Date created.
      |   Nov 30, 2012.  Edited mask because block was taking up too much space when placed into models.
  note: Simulink Sign block has three states (-1, 0, +1)
      | This block defines zero input as +1 sign.
  i : Inport
  Constant : Constant
  Constant1 : Constant  Value=-1
  Switch2 : Switch
  o : Outport
  wires:
  Constant/1 -> Switch2/1
  Constant1/1 -> Switch2/3
  i/1 -> Switch2/2
  Switch2/1 -> o/1

== system DevLib/Subsystems /Enabled Subsystem ==
  In1 : Inport
  Enable : EnablePort
  Out1 : Outport
  wires:
  In1/1 -> Out1/1

== system DevLib/Subsystems /Enabled and Triggered Subsystem ==
  In1 : Inport
  Enable : EnablePort
  Trigger : TriggerPort
  Out1 : Outport
  wires:
  In1/1 -> Out1/1

== system DevLib/Subsystems /Function-Call Subsystem ==
  In1 : Inport
  function : TriggerPort  TriggerType=function-call
  Out1 : Outport
  wires:
  In1/1 -> Out1/1

== system DevLib/Subsystems /Subsystem ==
  In1 : Inport
  Out1 : Outport
  wires:
  In1/1 -> Out1/1

== system DevLib/Subsystems /Triggered Subsystem ==
  In1 : Inport
  Trigger : TriggerPort
  Out1 : Outport
  wires:
  In1/1 -> Out1/1

== system DevLib/Subsystems /Variant Subsystem ==
  note: 1) Only subsystems can be added as variant choices at this level
      | 2) Blocks cannot be connected at this level as connectivity is
      | automatically determined at simulation, based on the active variant
  In1 : Inport
  Out1 : Outport

== system DevLib/Discrete/HP-CF Filter/1LP1-CF Filter ==
  note: Filter layout from spreadsheet
  note: This Subsystem represents a type 1LP1-CF Low-Pass filter with floating point math. Layout and nomenclature taken from Design Document authored by Mark Colosky.
  note: REVISIONS
      |   Feb 13, 2012.  Date created.
      |   Feb 17, 2012.  Conversion from Hz to Knum moved to Initialization tab of mask dialog box.
      |   Feb 20, 2012.  Parameterized 1/z block Initial Condition instead of hard-coded = 0.
      |   Jun 14, 2012.  Edited Icon to match other 1LP1-CF variants.
  In1 : Inport
  Constant : Constant  Value=Knum  OutDataTypeStr=Inherit: Inherit via back propagation
  Integer Delay : Delay  DelayLength=1  InitialCondition=IC  SampleTime=Ts
  Product1 : Product  RndMeth=Zero
  Sum : Sum  Inputs=|+-
  Sum1 : Sum  Inputs=|++
  Out : Outport
  wires:
  Sum1/1 -> Out/1, Integer Delay/1  "e"
  In1/1 -> Sum/1  "Unfiltered_Signal"
  Integer Delay/1 -> Sum/2, Sum1/2  "f"
  Product1/1 -> Sum1/1  "d"
  Constant/1 -> Product1/1
  Sum/1 -> Product1/2  "c"

== system DevLib/Discrete/HP-CF Filter /1LP1-CF Filter ==
  note: Filter layout from spreadsheet
  note: This Subsystem represents a type 1LP1-CF Low-Pass filter with floating point math.
      | Layout and nomenclature taken from Design Document authored by Mark Colosky.
  note: REVISIONS
      |   Feb 13, 2012.  Date created.
      |   Feb 17, 2012.  Conversion from Hz to Knum moved to Initialization tab of mask dialog box.
      |   Feb 20, 2012.  Parameterized 1/z block Initial Condition instead of hard-coded = 0.
      |   May 22, 2012.  Added external cutoff frequency signal.
  In1 : Inport
  KnHz : Inport  Port=2
  Constant : Constant  OutDataTypeStr=Inherit: Inherit via back propagation
  Constant1 : Constant  Value=-2*pi*Ts  OutDataTypeStr=Inherit: Inherit via back propagation
  Integer Delay : Delay  DelayLength=1  InitialCondition=IC  SampleTime=Ts
  Math Function : Math  SaturateOnIntegerOverflow=on
  Product1 : Product  RndMeth=Zero
  Product2 : Product  RndMeth=Zero
  Subtract : Sum  Inputs=+-
  Sum : Sum  Inputs=|+-
  Sum1 : Sum  Inputs=|++
  Out : Outport
  wires:
  Subtract/1 -> Product1/1
  Product2/1 -> Math Function/1
  KnHz/1 -> Product2/2
  Constant1/1 -> Product2/1
  Math Function/1 -> Subtract/2
  Constant/1 -> Subtract/1
  Sum1/1 -> Out/1, Integer Delay/1  "e"
  In1/1 -> Sum/1  "Unfiltered_Signal"
  Integer Delay/1 -> Sum/2, Sum1/2  "f"
  Product1/1 -> Sum1/1  "d"
  Sum/1 -> Product1/2  "c"
